simulink model "Simulation_MIMO_MPC_Dreitank_EKF"  (R2022b)
settings: Solver=ode3  StartTime=0.0  StopTime=150  MaxStep=0.01  RelTol=1e-3  EnableMultiTasking=on
PreLoadFcn:
  | A = [0 1;-1 -1];
  | B = [0 ; 1];
  | C = [1 0];
  | 
  | 
  | X0 = [0;0];
  | X_dot0 = [0;0];
  | Y0 = [0;];
  | U0 = [0];
  | 
  | X_AP = X0;
  | U_AP = U0;
  | Y_AP = Y0;
  | X_dot_AP = X_dot0;
undefined symbols (not defined in the file): EKF, MPC, N1, N2, Nu, T_MPC
libraries: UtilLib x1
settings Model: SimulationMode=rapid-accelerator  Creator=Matze  LastModifiedBy=vd818225
settings SolverCC: AlgebraicLoopSolver=TrustRegion
settings DataIOCC: SaveFormat=Array  SignalLoggingSaveFormat=ModelDataLogs  SaveOutput=off  SignalLogging=off  DSMLogging=off  SaveTime=off  ReturnWorkspaceOutputs=off
settings OptimizationCC: ExpressionDepthLimit=2147483647  LifeSpan=inf
settings DebuggingCC: UnderspecifiedInitializationDetection=Classic  MergeDetectMultiDrivingBlocksExec=none  SolverPrmCheckMsg=warning  InheritedTsInSrcMsg=none  FcnCallInpInsideContextMsg=warning  UnconnectedInputMsg=warning  UnconnectedOutputMsg=warning  UnconnectedLineMsg=warning  StateNameClashWarn=warning  SFUnexpectedBacktrackingDiag=warning  SFNoUnconditionalDefaultTransitionDiag=warning  SFExecutionAtInitializationDiag=none  SFMachineParentedDataDiag=warning  ArithmeticOperatorsInVariantConditions=warning
settings HardwareCC: ProdBitPerPointer=32  ProdBitPerSizeT=32  ProdBitPerPtrDiffT=32  ProdLargestAtomicFloat=None  ProdIntDivRoundTo=Undefined  ProdEndianess=Unspecified  ProdWordSize=32  ProdHWDeviceType=32-bit Generic
settings ModelReferenceCC: EnableRefExpFcnMdlSchedulingChecks=on  PropagateSignalLabelsOutOfModel=off
settings SFSimCC: SimUseLocalCustomCode=off  SimParseCustomCode=off  CustomCodeUndefinedFunction=UseInterfaceOnly
settings RTWCC: RTWUseLocalCustomCode=off  DLArmComputeVersion=19.05
settings CodeAppCC: StateflowObjectComments=on
settings GRTTargetCC: TargetLangStandard=C89/C90 (ANSI)  CombineOutputUpdateFcns=off  GRTInterface=on
settings ConfigComp: CovMetricSettings=dw  CovSaveCumulativeToWorkspaceVar=on  CovSaveSingleToWorkspaceVar=on  CovExternalEMLEnable=off

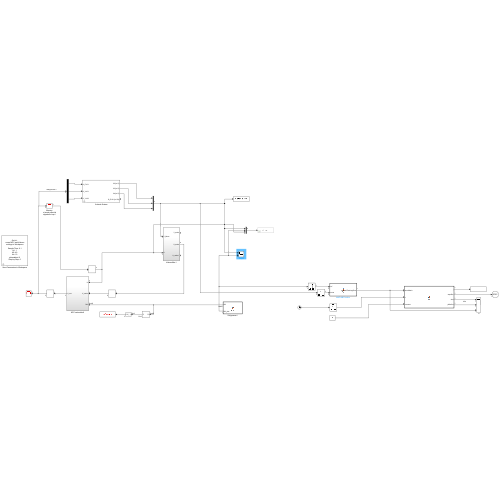
[thumbnail: Simulink's stored preview of the top-level diagram]
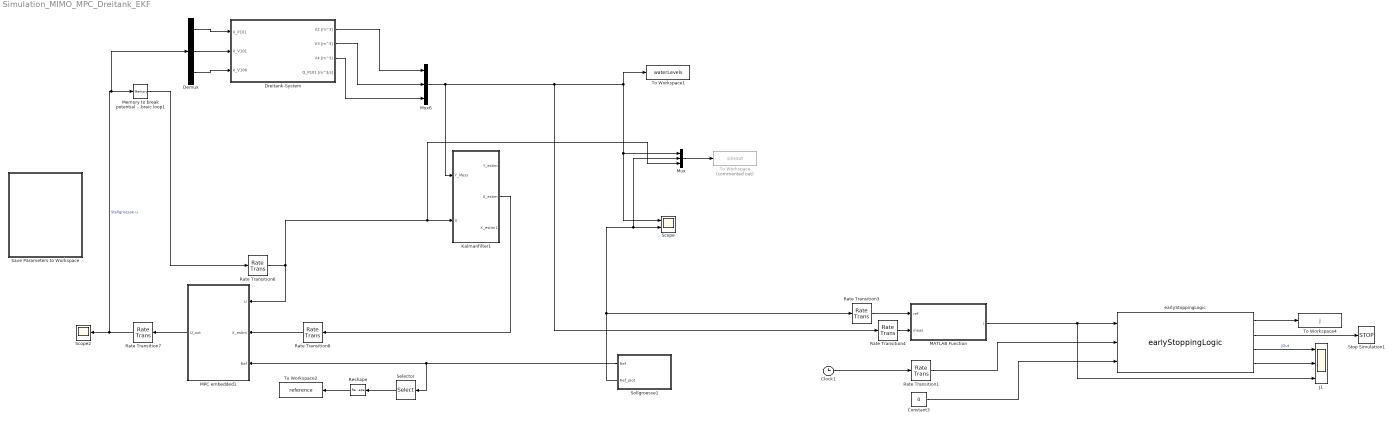
== system Simulation_MIMO_MPC_Dreitank_EKF ==
  Clock1 : Clock
  Constant3 : Constant  Value=0
  Demux : Demux  Outputs=3
  Dreitank-System : Subsystem  mask{B101_Volumen=80*10^-3, B102_Initial_Volumen=8*10^-3, B103_Initial_Volumen=6*10^-3, B104_Initial_Volumen=5*10^-3, Querschnitt_Rohr_B102_B103=600*10^-6, Querschnitt_Rohr_B103_B104=600*10^-6, Flaeche_Behaelter=0.029}
      mask prompts: B101_Volumen "Volumen im Behälter B101 in m^3"; B102_Initial_Volumen "Initialvolumen im Behälter B102 in m^3"; B103_Initial_Volumen "Initialvolumen im Behälter B103 in m^3"; B104_Initial_Volumen "Initialvolumen im Behälter B104 in m^3"; Querschnitt_Rohr_B102_B103 "Rohrquerschnitt zwischen Behälter B102 und B103 in m^2"; Querschnitt_Rohr_B103_B104 "Rohrquerschnitt zwischen Behälter B103 und B104 in m^2"; Flaeche_Behaelter "Fläche der Behälter in m^2"
  J1 : Scope  NumInputPorts=3
  Kalmanfilter1 : Subsystem
  MATLAB Function : MATLAB Function  TreatAsAtomicUnit=on
  MPC embedded1 : Subsystem
  Memory to break potential algrebraic loop1 : Memory
  Mux : Mux  Inputs=3
  Mux6 : Mux  Inputs=3
  Rate Transition1 : RateTransition  OutPortSampleTime=ESSettings.t_obj
  Rate Transition3 : RateTransition  OutPortSampleTime=ESSettings.t_obj
  Rate Transition4 : RateTransition  OutPortSampleTime=ESSettings.t_obj
  Rate Transition6 : RateTransition  OutPortSampleTimeOpt=Inherit  OutPortSampleTime=0.1
  Rate Transition7 : RateTransition  OutPortSampleTimeOpt=Inherit  OutPortSampleTime=0.1
  Rate Transition8 : RateTransition  OutPortSampleTimeOpt=Inherit  OutPortSampleTime=0.1
  Reshape : Reshape
  Save Parameters to Workspace : Subsystem  mask(Double-click open){T_MPC=0.1, N1=1, N2=40, Nu=10, PlotEnabled=off, StepByStep=off}
      mask prompts: T_MPC "Sample Time MPC/Kalman"; PlotEnabled "plot enabled"; StepByStep "Step-by-Step"
      mask init:
      | assignin('base','T_MPC',T_MPC);
      | assignin('base','N1',N1);
      | assignin('base','N2',N2);
      | assignin('base','Nu',Nu);
      | assignin('base','PlotEnabled',PlotEnabled);
      | assignin('base','StepByStep',StepByStep);
      mask Display:
      | disp(['On init: \n saves MPC and Kalman\n settings to Workspace\n\n'    ...
      |         'Sample Time: ' num2str(T_MPC) '\n'...
      |         'N1: ' num2str(N1) '\n'...
      |         'N2: ' num2str(N2) '\n'...
      |         'Nu: ' num2str(Nu) '\n'...
      |         'plotenabled: ' num2str(PlotEnabled) '\n'...
      |         'Step-by-Step: ' num2str(StepByStep) '\n'...
      | ]);
  Scope : Scope  NumInputPorts=2
  Scope2 : Scope
  Selector : Selector  NumberOfDimensions=2  InputPortWidth=3  IndexOptions=Index vector (dialog),Index vector (dialog)  Indices=[1:3],1  OutputSizes=1,1
  Sollgroesse1 : MATLAB Function  TreatAsAtomicUnit=on
  Stop Simulation1 : Stop
  To Workspace : ToWorkspace  Commented=on  VariableName=simout  SaveFormat=Timeseries  SampleTime=-1
  To Workspace1 : ToWorkspace  VariableName=waterLevels  SaveFormat=Structure With Time  SampleTime=0.1
  To Workspace2 : ToWorkspace  VariableName=reference  SaveFormat=Structure With Time  SampleTime=0.1
  To Workspace4 : ToWorkspace  VariableName=j  SaveFormat=Structure With Time  SampleTime=-1
  earlyStoppingLogic : UtilLib/earlyStoppingLogic  SystemSampleTime=-1  VariantActivationTime=update diagram  Latency=0  AutoFrameSizeCalculation=off
  wires:
  Sollgroesse1/1(Ref) -> Selector/1, MPC embedded1/3(Ref)
  Memory to break potential algrebraic loop1/1 -> Rate Transition6/1
  MPC embedded1/1(U_out) -> Rate Transition7/1
  Rate Transition6/1 -> MPC embedded1/1(U), Kalmanfilter1/2(U), Mux/3
  Rate Transition8/1 -> MPC embedded1/2(X_estim)
  Rate Transition7/1 -> Demux/1, Memory to break potential algrebraic loop1/1, Scope2/1  "Stellgroesse u"
  Mux/1 -> To Workspace/1
  Kalmanfilter1/2(X_estim) -> Rate Transition8/1
  Demux/1 -> Dreitank-System/1(U_P101)
  Demux/2 -> Dreitank-System/2("U_V101 ")
  Demux/3 -> Dreitank-System/3(U_V106)
  Dreitank-System/1(V2 [m^3]) -> Mux6/1
  Dreitank-System/2(V3 [m^3]) -> Mux6/2
  Dreitank-System/3(V4 [m^3]) -> Mux6/3
  Selector/1 -> Reshape/1
  Reshape/1 -> To Workspace2/1
  earlyStoppingLogic/4 -> J1/2
  earlyStoppingLogic/1 -> To Workspace4/1
  Rate Transition4/1 -> MATLAB Function/2(meas)
  MATLAB Function/1(j) -> J1/3, earlyStoppingLogic/1
  Rate Transition1/1 -> earlyStoppingLogic/2
  Clock1/1 -> Rate Transition1/1
  earlyStoppingLogic/2 -> Stop Simulation1/1
  Constant3/1 -> earlyStoppingLogic/3
  earlyStoppingLogic/3 -> J1/1  "JOut"
  Mux6/1 -> Kalmanfilter1/1(Y_Mess), Rate Transition4/1, Mux/1, Scope/1, To Workspace1/1
  Rate Transition3/1 -> MATLAB Function/1(ref)
  Sollgroesse1/2(Ref_plot) -> Rate Transition3/1, Mux/2, Scope/2

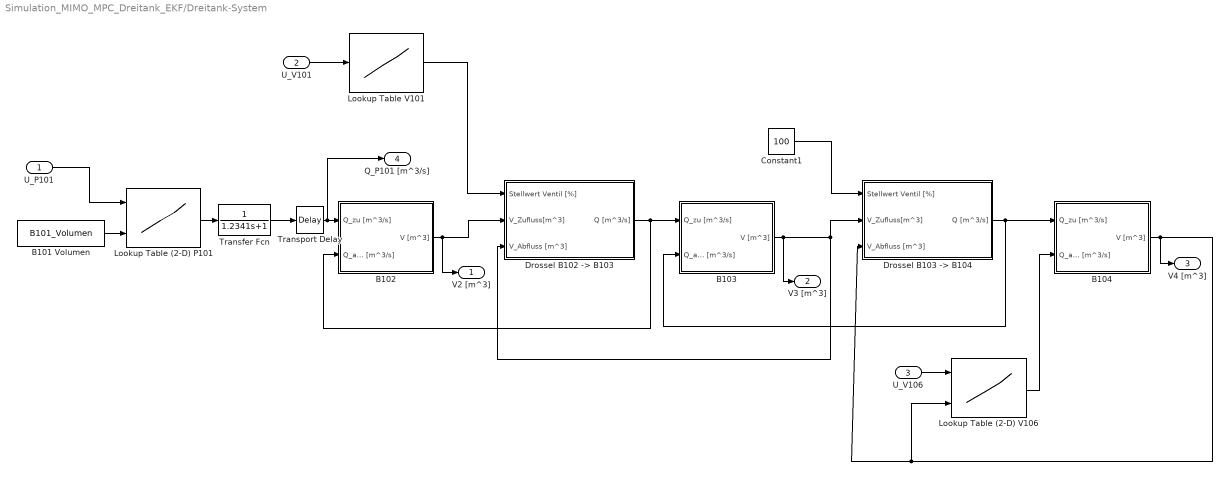
== system Simulation_MIMO_MPC_Dreitank_EKF/Dreitank-System ==
  U_P101 : Inport
  "U_V101 " : Inport  Port=2
  U_V106 : Inport  Port=3
  B101 Volumen : Constant  Value=B101_Volumen  OutDataTypeStr=double
  B102 : Subsystem  mask{Initial_Volumen=B102_Initial_Volumen}
      mask prompts: Initial_Volumen "Initialvolumen"
  B103 : Subsystem  mask{Initial_Volumen=B103_Initial_Volumen}
      mask prompts: Initial_Volumen "Initialvolumen"
  B104 : Subsystem  mask{Initial_Volumen=B104_Initial_Volumen}
      mask prompts: Initial_Volumen "Initialvolumen"
  Constant1 : Constant  Value=100
  "Drossel B102 -> B103" : Subsystem  mask{Querschnitt_Rohr=Querschnitt_Rohr_B102_B103, Flaeche_Behaelter=Flaeche_Behaelter}
      mask prompts: Querschnitt_Rohr "Querschnitt des Rohrs in m^2"; Flaeche_Behaelter "Flaeche_Behaelter in m^2"
  "Drossel B103 -> B104" : Subsystem  mask{Querschnitt_Rohr=Querschnitt_Rohr_B102_B103, Flaeche_Behaelter=Flaeche_Behaelter}
      mask prompts: Querschnitt_Rohr "Querschnitt des Rohrs in m^2"; Flaeche_Behaelter "Flaeche_Behaelter in m^2"
  Lookup Table (2-D) P101 : Lookup2D  RowIndex=[50,55,60,65,70,75,80,85,90,95,100]  ColumnIndex=[40,130]*10^-3  Table=reshape([0,0.0606,0.2450,0.3378,0.4184,0.5002,0.5801,0.6551,0.7138,0.7746,0.8206,0,0.2799,0.3497,0.4278,0.5053,0.5810,0.6481,0.7168,0.7695,0.8350,0.8786]*10^-3,11,2)  LookUpMeth=Interpolation-Use End Values  SaturateOnIntegerOverflow=off  InputSameDT=off
  Lookup Table (2-D) V106 : Lookup2D  RowIndex=[15,20,25,30,35,40,45,50,55,60,65,70,75,80,85]  ColumnIndex=[2,2.8,10]*10^-3  Table=reshape([0,0,0,0,0,0,0,0,0,0,0,0,0,0,0,0,0.032,0.097,0.179,0.262,0.361,0.475,0.604,0.902,1.089,1.318,1.536,1.685,1.853,2.029,0,0.032,0.097,0.179,0.262,0.361,0.475,0.604,0.902,1.089,1.318,1.536,1.685,1.853,2.029]*10^-3,15,3)  LookUpMeth=Interpolation-Use End Values  SaturateOnIntegerOverflow=off  InputSameDT=off
  Lookup Table V101 : Lookup  InputValues=[0,20,25,30,35,40,45,50,55,60,65,70,75,80,85,90,100]  Table=[100,96,90,88,84,76,68,60,49,41,34,27,22,19,16,12,0]  LookUpMeth=Interpolation-Use End Values  SaturateOnIntegerOverflow=off
  Transfer Fcn : TransferFcn  Denominator=[1.2341 1]
  Transport Delay : TransportDelay  DelayTime=1.1
  V2 [m^3] : Outport
  V3 [m^3] : Outport  Port=2
  V4 [m^3] : Outport  Port=3
  Q_P101 [m^3/s] : Outport  Port=4
  wires:
  "Drossel B103 -> B104"/1(Q [m^3/s]) -> B104/1(Q_zu [m^3/s]), B103/2(Q_ab [m^3/s])
  "Drossel B102 -> B103"/1(Q [m^3/s]) -> B102/2(Q_ab [m^3/s]), B103/1(Q_zu [m^3/s])
  B101 Volumen/1 -> Lookup Table (2-D) P101/2
  B103/1(V [m^3]) -> "Drossel B103 -> B104"/2(V_Zufluss[m^3]), "Drossel B102 -> B103"/3(V_Abfluss [m^3]), V3 [m^3]/1
  U_P101/1 -> Lookup Table (2-D) P101/1
  U_V106/1 -> Lookup Table (2-D) V106/1
  Lookup Table V101/1 -> "Drossel B102 -> B103"/1(Stellwert Ventil [%])
  Lookup Table (2-D) V106/1 -> B104/2(Q_ab [m^3/s])
  B102/1(V [m^3]) -> V2 [m^3]/1, "Drossel B102 -> B103"/2(V_Zufluss[m^3])
  "U_V101 "/1 -> Lookup Table V101/1
  B104/1(V [m^3]) -> Lookup Table (2-D) V106/2, "Drossel B103 -> B104"/3(V_Abfluss [m^3]), V4 [m^3]/1
  Constant1/1 -> "Drossel B103 -> B104"/1(Stellwert Ventil [%])
  Transfer Fcn/1 -> Transport Delay/1
  Transport Delay/1 -> Q_P101 [m^3/s]/1, B102/1(Q_zu [m^3/s])
  Lookup Table (2-D) P101/1 -> Transfer Fcn/1

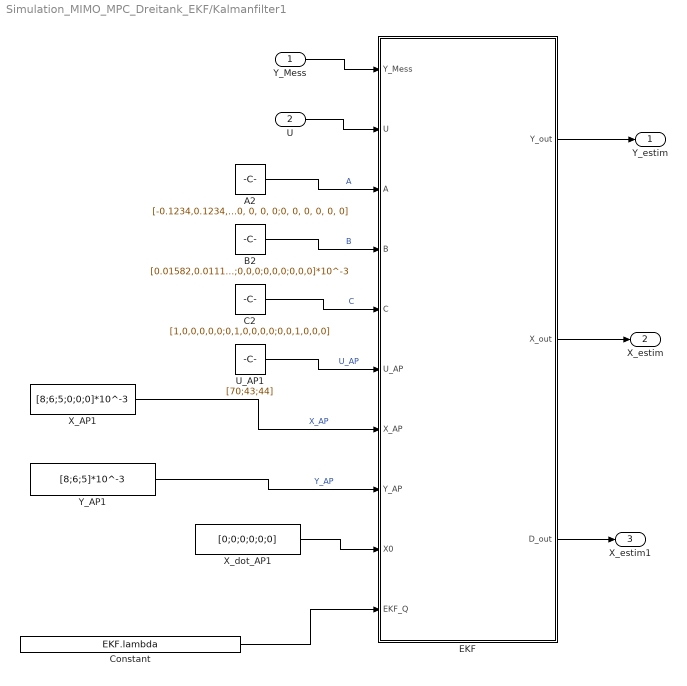
== system Simulation_MIMO_MPC_Dreitank_EKF/Kalmanfilter1 ==
  Y_Mess : Inport
  U : Inport  Port=2
  A2 : Constant  Value=[-0.1234,0.1234,0, 0.025,0,0;0.1234,-0.3702,0.2468, 0,0.025,0 ;0,0.2468,-0.2468, 0,0,0.025; 0, 0, 0, 0, 0, 0;0, 0, 0, 0, 0, 0;0, 0, 0, 0, 0, 0]  VectorParams1D=off
  B2 : Constant  Value=[0.01582,0.01117,0;0,-0.01117,0;0,0,-0.0228;0,0,0;0,0,0;0,0,0]*10^-3  VectorParams1D=off
  C2 : Constant  Value=[1,0,0,0,0,0;0,1,0,0,0,0;0,0,1,0,0,0]  VectorParams1D=off
  Constant : Constant  Value=EKF.lambda
  EKF : MATLAB Function  TreatAsAtomicUnit=on
  U_AP1 : Constant  Value=[70;43;44]  VectorParams1D=off
  X_AP1 : Constant  Value=[8;6;5;0;0;0]*10^-3  VectorParams1D=off
  X_dot_AP1 : Constant  Value=[0;0;0;0;0;0]  VectorParams1D=off
  Y_AP1 : Constant  Value=[8;6;5]*10^-3  VectorParams1D=off
  Y_estim : Outport  VectorParamsAs1DForOutWhenUnconnected=off
  X_estim : Outport  Port=2  VectorParamsAs1DForOutWhenUnconnected=off
  X_estim1 : Outport  Port=3  VectorParamsAs1DForOutWhenUnconnected=off
  wires:
  EKF/1(Y_out) -> Y_estim/1
  U/1 -> EKF/2(U)
  Y_Mess/1 -> EKF/1(Y_Mess)
  EKF/2(X_out) -> X_estim/1
  EKF/3(D_out) -> X_estim1/1
  C2/1 -> EKF/5(C)  "C"
  A2/1 -> EKF/3(A)  "A"
  B2/1 -> EKF/4(B)  "B"
  Y_AP1/1 -> EKF/8(Y_AP)  "Y_AP"
  U_AP1/1 -> EKF/6(U_AP)  "U_AP"
  X_dot_AP1/1 -> EKF/9(X0)
  X_AP1/1 -> EKF/7(X_AP)  "X_AP"
  Constant/1 -> EKF/10(EKF_Q)

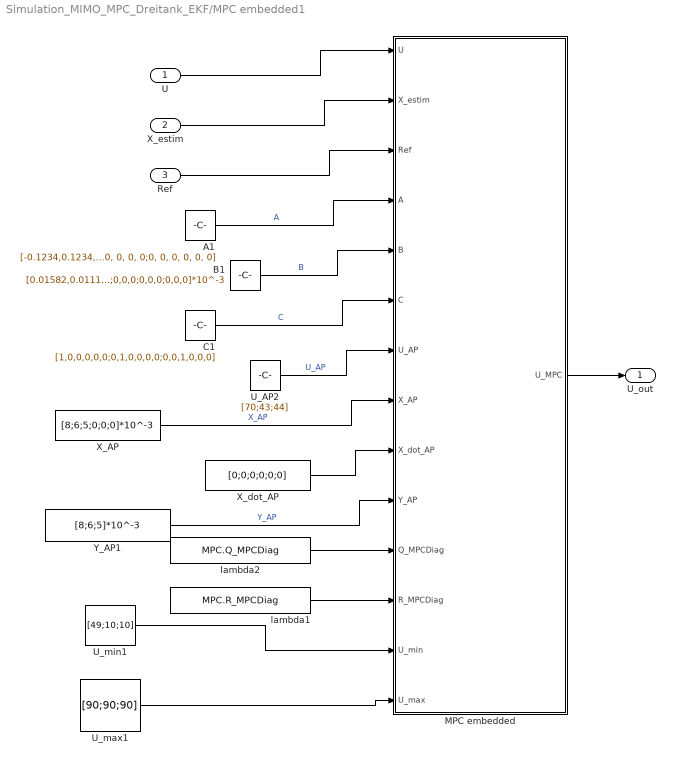
== system Simulation_MIMO_MPC_Dreitank_EKF/MPC embedded1 ==
  U : Inport
  X_estim : Inport  Port=2
  Ref : Inport  Port=3
  A1 : Constant  Value=[-0.1234,0.1234,0, 0.025,0,0;0.1234,-0.3702,0.2468, 0,0.025,0 ;0,0.2468,-0.2468, 0,0,0.025; 0, 0, 0, 0, 0, 0;0, 0, 0, 0, 0, 0;0, 0, 0, 0, 0, 0]  VectorParams1D=off
  B1 : Constant  Value=[0.01582,0.01117,0;0,-0.01117,0;0,0,-0.0228;0,0,0;0,0,0;0,0,0]*10^-3  VectorParams1D=off
  C1 : Constant  Value=[1,0,0,0,0,0;0,1,0,0,0,0;0,0,1,0,0,0]  VectorParams1D=off
  MPC embedded : MATLAB Function  TreatAsAtomicUnit=on
  U_AP2 : Constant  Value=[70;43;44]  VectorParams1D=off
  U_max1 : Constant  Value=[90;90;90]  VectorParams1D=off
  U_min1 : Constant  Value=[49;10;10]  VectorParams1D=off
  X_AP : Constant  Value=[8;6;5;0;0;0]*10^-3  VectorParams1D=off
  X_dot_AP : Constant  Value=[0;0;0;0;0;0]  VectorParams1D=off
  Y_AP1 : Constant  Value=[8;6;5]*10^-3  VectorParams1D=off
  lambda1 : Constant  Value=MPC.R_MPCDiag  VectorParams1D=off
  lambda2 : Constant  Value=MPC.Q_MPCDiag  VectorParams1D=off
  U_out : Outport  VectorParamsAs1DForOutWhenUnconnected=off
  wires:
  B1/1 -> MPC embedded/5(B)  "B"
  C1/1 -> MPC embedded/6(C)  "C"
  lambda2/1 -> MPC embedded/11(Q_MPCDiag)
  Y_AP1/1 -> MPC embedded/10(Y_AP)  "Y_AP"
  U_max1/1 -> MPC embedded/14(U_max)
  A1/1 -> MPC embedded/4(A)  "A"
  X_dot_AP/1 -> MPC embedded/9(X_dot_AP)
  MPC embedded/1(U_MPC) -> U_out/1
  X_AP/1 -> MPC embedded/8(X_AP)  "X_AP"
  U_AP2/1 -> MPC embedded/7(U_AP)  "U_AP"
  X_estim/1 -> MPC embedded/2(X_estim)
  U/1 -> MPC embedded/1(U)
  Ref/1 -> MPC embedded/3(Ref)
  U_min1/1 -> MPC embedded/13(U_min)
  lambda1/1 -> MPC embedded/12(R_MPCDiag)

== system Simulation_MIMO_MPC_Dreitank_EKF/Save Parameters to Workspace ==

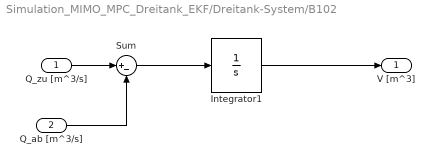
== system Simulation_MIMO_MPC_Dreitank_EKF/Dreitank-System/B102 ==
  Q_zu [m^3/s] : Inport
  Q_ab [m^3/s] : Inport  Port=2
  Integrator1 : Integrator  InitialCondition=Initial_Volumen  LimitOutput=on  UpperSaturationLimit=10*10^-3  LowerSaturationLimit=0  ContinuousStateAttributes='Volumen_B102'
  Sum : Sum  Inputs=|+-
  V [m^3] : Outport
  wires:
  Q_ab [m^3/s]/1 -> Sum/2
  Q_zu [m^3/s]/1 -> Sum/1
  Integrator1/1 -> V [m^3]/1
  Sum/1 -> Integrator1/1

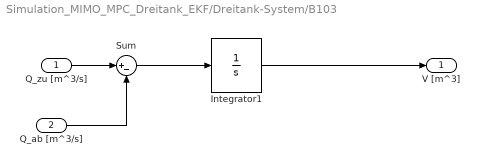
== system Simulation_MIMO_MPC_Dreitank_EKF/Dreitank-System/B103 ==
  Q_zu [m^3/s] : Inport
  Q_ab [m^3/s] : Inport  Port=2
  Integrator1 : Integrator  InitialCondition=Initial_Volumen  LimitOutput=on  UpperSaturationLimit=10*10^-3  LowerSaturationLimit=0  ContinuousStateAttributes='Volumen_B102'
  Sum : Sum  Inputs=|+-
  V [m^3] : Outport
  wires:
  Q_ab [m^3/s]/1 -> Sum/2
  Q_zu [m^3/s]/1 -> Sum/1
  Integrator1/1 -> V [m^3]/1
  Sum/1 -> Integrator1/1

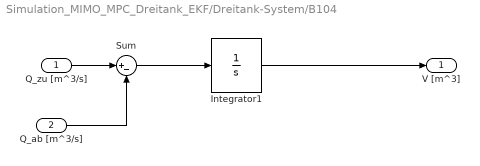
== system Simulation_MIMO_MPC_Dreitank_EKF/Dreitank-System/B104 ==
  Q_zu [m^3/s] : Inport
  Q_ab [m^3/s] : Inport  Port=2
  Integrator1 : Integrator  InitialCondition=Initial_Volumen  LimitOutput=on  UpperSaturationLimit=10*10^-3  LowerSaturationLimit=0  ContinuousStateAttributes='Volumen_B102'
  Sum : Sum  Inputs=|+-
  V [m^3] : Outport
  wires:
  Sum/1 -> Integrator1/1
  Integrator1/1 -> V [m^3]/1
  Q_zu [m^3/s]/1 -> Sum/1
  Q_ab [m^3/s]/1 -> Sum/2

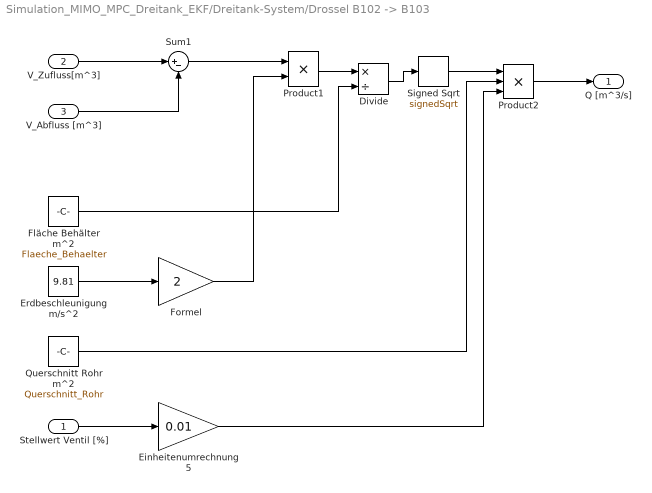
== system Simulation_MIMO_MPC_Dreitank_EKF/Dreitank-System/Drossel B102 -> B103 ==
  Stellwert Ventil [%] : Inport
  V_Zufluss[m^3] : Inport  Port=2
  V_Abfluss [m^3] : Inport  Port=3
  Divide : Product  Inputs=*/
  Einheitenumrechnung 5 : Gain  Gain=0.01
  Erdbeschleunigung m/s^2 : Constant  Value=9.81  OutDataTypeStr=double
  Fläche Behälter m^2 : Constant  Value=Flaeche_Behaelter  OutDataTypeStr=double
  Formel : Gain  Gain=2
  Product1 : Product  RndMeth=Zero
  Product2 : Product  Inputs=3  RndMeth=Zero
  Querschnitt Rohr m^2 : Constant  Value=Querschnitt_Rohr  OutDataTypeStr=double
  Signed Sqrt : Sqrt  Operator=signedSqrt
  Sum1 : Sum  Inputs=|+-
  Q [m^3/s] : Outport
  wires:
  Fläche Behälter m^2/1 -> Divide/2
  Divide/1 -> Signed Sqrt/1
  Product1/1 -> Divide/1
  Formel/1 -> Product1/2
  Sum1/1 -> Product1/1
  V_Abfluss [m^3]/1 -> Sum1/2
  V_Zufluss[m^3]/1 -> Sum1/1
  Product2/1 -> Q [m^3/s]/1
  Einheitenumrechnung 5/1 -> Product2/3
  Stellwert Ventil [%]/1 -> Einheitenumrechnung 5/1
  Querschnitt Rohr m^2/1 -> Product2/2
  Signed Sqrt/1 -> Product2/1
  Erdbeschleunigung m/s^2/1 -> Formel/1

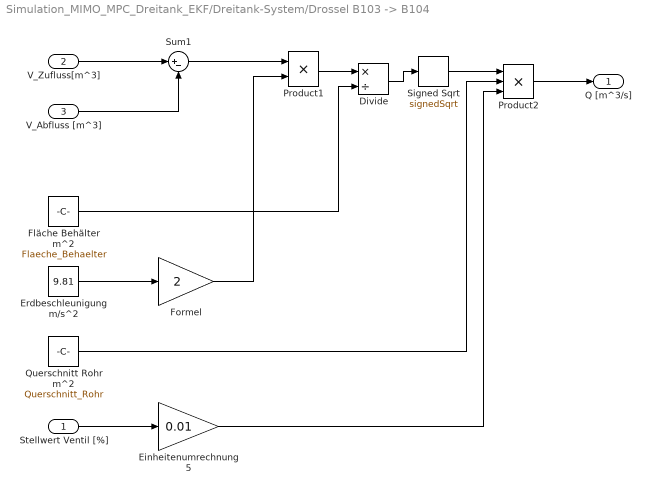
== system Simulation_MIMO_MPC_Dreitank_EKF/Dreitank-System/Drossel B103 -> B104 ==
  Stellwert Ventil [%] : Inport
  V_Zufluss[m^3] : Inport  Port=2
  V_Abfluss [m^3] : Inport  Port=3
  Divide : Product  Inputs=*/
  Einheitenumrechnung 5 : Gain  Gain=0.01
  Erdbeschleunigung m/s^2 : Constant  Value=9.81  OutDataTypeStr=double
  Fläche Behälter m^2 : Constant  Value=Flaeche_Behaelter  OutDataTypeStr=double
  Formel : Gain  Gain=2
  Product1 : Product  RndMeth=Zero
  Product2 : Product  Inputs=3  RndMeth=Zero
  Querschnitt Rohr m^2 : Constant  Value=Querschnitt_Rohr  OutDataTypeStr=double
  Signed Sqrt : Sqrt  Operator=signedSqrt
  Sum1 : Sum  Inputs=|+-
  Q [m^3/s] : Outport
  wires:
  Erdbeschleunigung m/s^2/1 -> Formel/1
  Signed Sqrt/1 -> Product2/1
  Querschnitt Rohr m^2/1 -> Product2/2
  Stellwert Ventil [%]/1 -> Einheitenumrechnung 5/1
  Einheitenumrechnung 5/1 -> Product2/3
  Product2/1 -> Q [m^3/s]/1
  V_Zufluss[m^3]/1 -> Sum1/1
  V_Abfluss [m^3]/1 -> Sum1/2
  Sum1/1 -> Product1/1
  Formel/1 -> Product1/2
  Product1/1 -> Divide/1
  Divide/1 -> Signed Sqrt/1
  Fläche Behälter m^2/1 -> Divide/2

== matlab function Simulation_MIMO_MPC_Dreitank_EKF/MATLAB Function ==
  data: ref input; j output; meas input
function j  = fcn(ref, meas)
j = sum(abs(ref-meas));
end

== matlab function Simulation_MIMO_MPC_Dreitank_EKF/Kalmanfilter1/EKF ==
  settings: updateMethod=DISCRETE  sampleTime=T_MPC
  data: Y_out output; Y_Mess input; U input; A input; B input; C input; U_AP input; X_AP input; Y_AP input; X0 input; EKF_Q input; T_MPC parameter; X_out output; D_out output
function [Y_out, X_out, D_out]  = EKF(Y_Mess,U, A,B,C,U_AP,X_AP, Y_AP, X0,EKF_Q, T_MPC) %#codegen
%%%%%%%%%%%%%%%%%%%%%%%%%%%%%%%%%%%%%%%%%%%%%%%%%%%%%%%%%%%%%%%%%%%%%%%%%%%%%%
% Einfaches Extended Kalmanfilter zur Bestimmung der Zustände am Ende des aktuellen
% Zeitschrittes.
%
% A,B,C: Linearisierte Systemdarstellung
% U_AP, X_AP, Y_AP: Absolutgrößen am Arbeitspunkt (Linearisierung)
% X_dot_AP:         Ableitung des Zustandes am Arbeitspunkt (= 0 für
%                   stationären Arbeitspunkt
% T_MPC:            Abtastrate
%
% Y_Mess: Messgrößenvektor
% X0    : Initialisierungszustand
%
% X_out: Prädierter Zustand am Ende des aktuellen Zeitschrittes
% Y_out: Prädizierte Ausgangsgröße am Ende des aktuellen Zeitschrittes
%
%%%%%%%%%%%%%%%%%%%%%%%%%%%%%%%%%%%%%%%%%%%%%%%%%%%%%%%%%%%%%%%%%%%%%%%%%%%%%%
% Empfohlener Artikel für erste Kalman-Kontakte:
% C. Baumann, "Das Kalman Filter wird 50"
% http://www.convict.lu/htm/rob/Das%20Kalman%20Filter%20wird%2050_v_1.4.pdf
%%%%%%%%%%%%%%%%%%%%%%%%%%%%%%%%%%%%%%%%%%%%%%%%%%%%%%%%%%%%%%%%%%%%%%%%%%%%%%

%%%%%%%%%%%%%%%%%%%%%%%%%%%%%%%%%%%%%%%%%%%%%%%%%%%%%%%%%%%%%%%%%%%%%%%%%%%%%%
%% Zeitkontiunierlich->Zeitdiskret
%%%%%%%%%%%%%%%%%%%%%%%%%%%%%%%%%%%%%%%%%%%%%%%%%%%%%%%%%%%%%%%%%%%%%%%%%%%%%%
[AD, BD, CD]            = Continuous2Discrete(A,B,C,T_MPC);

%%%%%%%%%%%%%%%%%%%%%%%%%%%%%%%%%%%%%%%%%%%%%%%%%%%%%%%%%%%%%%%%%%%%%%%%%%%%%%
%% Initialisierung Zustände im Filter
%%%%%%%%%%%%%%%%%%%%%%%%%%%%%%%%%%%%%%%%%%%%%%%%%%%%%%%%%%%%%%%%%%%%%%%%%%%%%%
persistent X P
if isempty(X)
    X = X0;
    P =  diag(ones(1,size(AD,1)),0 );
end

%%%%%%%%%%%%%%%%%%%%%%%%%%%%%%%%%%%%%%%%%%%%%%%%%%%%%%%%%%%%%%%%%%%%%%%%%%%%%%
%% Umwandlung in Relativgroessen:
%%%%%%%%%%%%%%%%%%%%%%%%%%%%%%%%%%%%%%%%%%%%%%%%%%%%%%%%%%%%%%%%%%%%%%%%%%%%%%
x = X-X_AP;
u = U-U_AP;

%%%%%%%%%%%%%%%%%%%%%%%%%%%%%%%%%%%%%%%%%%%%%%%%%%%%%%%%%%%%%%%%%%%%%%%%%%%%%%
%% Kovarianzmatritzen:
%%%%%%%%%%%%%%%%%%%%%%%%%%%%%%%%%%%%%%%%%%%%%%%%%%%%%%%%%%%%%%%%%%%%%%%%%%%%%%
% Prozessrauschen:
Q = diag(EKF_Q);%diag([1 1 1 10^2 5^2 5^2]);
% Messrauschen:
R = diag(ones(1,size(CD,1)))*10^-2;
%%%%%%%%%%%%%%%%%%%%%%%%%%%%%%%%%%%%%%%%%%%%%%%%%%%%%%%%%%%%%%%%%%%%%%%%%%%%%%%
%% Korrekturschritt
%%%%%%%%%%%%%%%%%%%%%%%%%%%%%%%%%%%%%%%%%%%%%%%%%%%%%%%%%%%%%%%%%%%%%%%%%%%%%%%
MI = CD*P*CD' + R;
K = P*CD'/MI;
deltax = K*(Y_Mess - (Y_AP+CD*x));
x = x+deltax;
P = (eye(size(P)) - K*CD)*P;

%%%%%%%%%%%%%%%%%%%%%%%%%%%%%%%%%%%%%%%%%%%%%%%%%%%%%%%%%%%%%%%%%%%%%%%%%%%%%%%
%% Prädiktionsschritt (hier linear mit aktuellem Modell)
%%%%%%%%%%%%%%%%%%%%%%%%%%%%%%%%%%%%%%%%%%%%%%%%%%%%%%%%%%%%%%%%%%%%%%%%%%%%%%%
x = AD*x+BD*u;   
P = AD*P*AD'+Q;

%%%%%%%%%%%%%%%%%%%%%%%%%%%%%%%%%%%%%%%%%%%%%%%%%%%%%%%%%%%%%%%%%%%%%%%%%%%%%%
%% Umwandlung in Absolutgroessen:
%%%%%%%%%%%%%%%%%%%%%%%%%%%%%%%%%%%%%%%%%%%%%%%%%%%%%%%%%%%%%%%%%%%%%%%%%%%%%%
X = X_AP+x;

%%%%%%%%%%%%%%%%%%%%%%%%%%%%%%%%%%%%%%%%%%%%%%%%%%%%%%%%%%%%%%%%%%%%%%%%%%%%%%%
%% Ausgabe Zustand für nächsten Zeitschritt
%%%%%%%%%%%%%%%%%%%%%%%%%%%%%%%%%%%%%%%%%%%%%%%%%%%%%%%%%%%%%%%%%%%%%%%%%%%%%%%
X_out = X;
Y_out = Y_AP+CD*x;
D_out = P;
end

== matlab function Simulation_MIMO_MPC_Dreitank_EKF/MPC embedded1/MPC embedded ==
  settings: updateMethod=DISCRETE  sampleTime=T_MPC
  data: U input; X_estim input; Ref input; A input; B input; C input; U_AP input; X_AP input; X_dot_AP input; Y_AP input; T_MPC parameter; N1 parameter; N2 parameter; Nu parameter; Q_MPCDiag input; R_MPCDiag input; U_min input; U_max input; U_MPC output
function U_MPC   = MPC_embedded(U,X_estim, Ref, A,B,C,U_AP,X_AP, X_dot_AP, Y_AP,T_MPC, N1, N2, Nu,Q_MPCDiag,R_MPCDiag,U_min, U_max) %#codegen
%%%%%%%%%%%%%%%%%%%%%%%%%%%%%%%%%%%%%%%%%%%%%%%%%%%%%%%%%%%%%%%%%%%%%%%%%
% Gedacht als Referenz-/Beispielimplementierung RT-Skript 
% Im Wesentlichen Umsetzung aus RT-Skript.
% Erweiterung:
%   -Beschränkung Absolutwert Eingangsgroessen
%   -Instationäre Arbeitspunkte möglich
% Verbesserungsvorschläge gerne an RE

%%%%%%%%%%%%%%%%%%%%%%%%%%%%%%%%%%%%%%%%%%%%%%%%%%%%%%%%%%%%%%%%%%%%%%%%%
% Eingangsgrößen:
% U          : Aktueller Absolutert der Stellgröße an der Anlage
% X_estim    : Geschätzer Absolutwert des Zustands am Ende des Zeitschrittes
% Ref        : Sollwertvorgabe (absolut), für jede Regelgröße eine Zeile, passend zum
%              gewählten Prädiktionshorizont
%%%%%%%%%%%%%%%%%%%%%%%%%%%%%%%%%%%%%%%%%%%%%%%%%%%%%%%%%%%%%%%%%%%%%%%%%
% Linearisierte Systembeschreibung:
% A          : Systemmatrix linearisiertes System (kontinuierlich)
% B          : Einfangsmatrix linearisiertes System (kontinuierlich)
% C          : Ausgangsmatrix linearisiertes System (kontinuierlich)
% U_AP       : Stellgröße im Arbeitspunkt
% X_AP       : Zustand im Arbeitspunkt
% X_dot_AP   : Ableitung Zustand im Arbeitspunkt (0 für stationäre Arbeitspunkte) 
% Y_AP       : Ausgang im Arbeitspunkt
%%%%%%%%%%%%%%%%%%%%%%%%%%%%%%%%%%%%%%%%%%%%%%%%%%%%%%%%%%%%%%%%%%%%%%%%%
% MPC-Parameter
% T_MPC      : Abtastschritt
% N1         : unterer Prädiktionshorizont
% N2         : oberer Prädiktionshorizont
% Nu         : Stellhorizont
% lambda_MPC : relative Gewichtung Stellgrößenänderung
% U_min      : Minimalwert Stellgröße (Beschränkung)
% U_max      : Maximalwert Stellgröße (Beschränkung)
%%%%%%%%%%%%%%%%%%%%%%%%%%%%%%%%%%%%%%%%%%%%%%%%%%%%%%%%%%%%%%%%%%%%%%%%%
% Dokumentation und Plot:
% PlotEnabled: Darstellung Werte in Plot
% StepByStep : Pause nach Plot
% Y_doku     : Tatsächlicher Wert Ausgangsgröße (zum Vergleich in Plot)
% currentTime: Simulationszeit für Dokumentation
%%%%%%%%%%%%%%%%%%%%%%%%%%%%%%%%%%%%%%%%%%%%%%%%%%%%%%%%%%%%%%%%%%%%%%%%%


%%%%%%%%%%%%%%%%%%%%%%%%%%%%%%%%%%%%%%%%%%%%%%%%%%%%%%%%%%%%%%%%%%%%%%%%%
%% Berechnung diskrete Zustandsraumdarstellung
%%%%%%%%%%%%%%%%%%%%%%%%%%%%%%%%%%%%%%%%%%%%%%%%%%%%%%%%%%%%%%%%%%%%%%%%%
tic
[AD, BD, CD]        = Continuous2Discrete(A,B,C,T_MPC);

%%%%%%%%%%%%%%%%%%%%%%%%%%%%%%%%%%%%%%%%%%%%%%%%%%%%%%%%%%%%%%%%%%%%%%%%%
%% Generierung MPC-Matritzen
%%%%%%%%%%%%%%%%%%%%%%%%%%%%%%%%%%%%%%%%%%%%%%%%%%%%%%%%%%%%%%%%%%%%%%%%%
[MCA, MCAB,MPhi] = GenerateMPCMatrices(AD,BD,CD, N1, N2, Nu);

%%%%%%%%%%%%%%%%%%%%%%%%%%%%%%%%%%%%%%%%%%%%%%%%%%%%%%%%%%%%%%%%%%%%%%%%%
%% Zwischenvariablen als Hilfestellung 
%%%%%%%%%%%%%%%%%%%%%%%%%%%%%%%%%%%%%%%%%%%%%%%%%%%%%%%%%%%%%%%%%%%%%%%%%
AnzahlStellgroessen = size(BD,2);
AnzahlRegelgroessen = size(CD,1);
Horizontlaenge      = N2-N1+1;

%%%%%%%%%%%%%%%%%%%%%%%%%%%%%%%%%%%%%%%%%%%%%%%%%%%%%%%%%%%%%%%%%%%%%%%%%
%% Umsortieren Referenzggröße auf Vektorform:
%%%%%%%%%%%%%%%%%%%%%%%%%%%%%%%%%%%%%%%%%%%%%%%%%%%%%%%%%%%%%%%%%%%%%%%%%
Ref_vec = reshape(Ref, size(Ref,1)*size(Ref,2),1);

%%%%%%%%%%%%%%%%%%%%%%%%%%%%%%%%%%%%%%%%%%%%%%%%%%%%%%%%%%%%%%%%%%%%%%%%%
%% Umrechnung Absolutgrößen in Größen bezogen auf Arbeitspunkt
%%%%%%%%%%%%%%%%%%%%%%%%%%%%%%%%%%%%%%%%%%%%%%%%%%%%%%%%%%%%%%%%%%%%%%%%%
xk      = X_estim-X_AP;                                 %Zustand
u_km1    = U - U_AP;                                    %Stellgröße aktuell
r       = Ref_vec - repmat(Y_AP,Horizontlaenge,1);      %Sollwert
%%%%%%%%%%%%%%%%%%%%%%%%%%%%%%%%%%%%%%%%%%%%%%%%%%%%%%%%%%%%%%%%%%%%%%%%%
%% Freie Regelgröße (Skript Gl. 10.14) mit Erweiterung um instationären Term
%%%%%%%%%%%%%%%%%%%%%%%%%%%%%%%%%%%%%%%%%%%%%%%%%%%%%%%%%%%%%%%%%%%%%%%%%
%f = MCA*xk + X_estim(4)+MCAB*u_km1 ;
f = MCA*xk +MCAB*u_km1 ;


%%%%%%%%%%%%%%%%%%%%%%%%%%%%%%%%%%%%%%%%%%%%%%%%%%%%%%%%%%%%%%%%%%%%%%%%%
%% Freie Regelabweichung:
%%%%%%%%%%%%%%%%%%%%%%%%%%%%%%%%%%%%%%%%%%%%%%%%%%%%%%%%%%%%%%%%%%%%%%%%%
e = f-r ;

%%%%%%%%%%%%%%%%%%%%%%%%%%%%%%%%%%%%%%%%%%%%%%%%%%%%%%%%%%%%%%%%%%%%%%%%%
%% Wichtungsmatritzen
%%%%%%%%%%%%%%%%%%%%%%%%%%%%%%%%%%%%%%%%%%%%%%%%%%%%%%%%%%%%%%%%%%%%%%%%%
%Q_MPC = eye(AnzahlRegelgroessen*Horizontlaenge);  % Für jeden vorhergesagten Wert des Ausgangs und für jeden Zeitschritt
Q_MPC = diag(repmat([Q_MPCDiag],1,Horizontlaenge));  % Für jeden vorhergesagten Wert des Ausgangs und für jeden Zeitschritt
%R_MPC = eye(AnzahlStellgroessen*Nu)*lambda_MPC;   %Für jeden vorhergesagten Wert der Stellgrößenänderung und für jeden Zeitschritt
R_MPC = diag(repmat([R_MPCDiag],1,Nu));
%%%%%%%%%%%%%%%%%%%%%%%%%%%%%%%%%%%%%%%%%%%%%%%%%%%%%%%%%%%%%%%%%%%%%%%%%
%% Aufstellen Optimierungsproblem
%%%%%%%%%%%%%%%%%%%%%%%%%%%%%%%%%%%%%%%%%%%%%%%%%%%%%%%%%%%%%%%%%%%%%%%%%
% Erstelle Problem der Form:
% Minimiere 1/2*x'*H_qp*x + f_qp'*x unter der Bedingung: A_qp*x <=b_qp
%%%%%%%%%%%%%%%%%%%%%%%%%%%%%%%%%%%%%%%%%%%%%%%%%%%%%%%%%%%%%%%%%%%%%%%%%
H_qp = (MPhi'*Q_MPC'*MPhi+R_MPC);
f_qp =  (e'*Q_MPC*MPhi)';
%%%%%%%%%%%%%%%%%%%%%%%%%%%%%%%%%%%%%%%%%%%%%%%%%%%%%%%%%%%%%%%%%%%%%%%%%
%%%%%%%%%%%%%%%%%%%%%%%%%%%%%%%%%%%%%%%%%%%%%%%%%%%%%%%%%%%%%%%%%%%%%%%%%
% Für Begrenzung (Hier Beispiel Absolutwert Stellgroesse)
% Matrix für Berechnung von Uabs
%%%%%%%%%%%%%%%%%%%%%%%%%%%%%%%%%%%%%%%%%%%%%%%%%%%%%%%%%%%%%%%%%%%%%%%%%
MDiag = zeros(AnzahlStellgroessen*Nu);
for Horiz = 1:Nu
    for Stellg = 1:AnzahlStellgroessen
        for iHoriz = 1:Horiz
            MDiag((Horiz-1)*AnzahlStellgroessen+1+(Stellg-1),...
                (Stellg-1) +1+(iHoriz-1)*AnzahlStellgroessen) = 1;
        end
    end
end
%%%%%%%%%%%%%%%%%%%%%%%%%%%%%%%%%%%%%%%%%%%%%%%%%%%%%%%%%%%%%%%%%%%%%%%%%
A_qp = [MDiag; -MDiag];
b_qp = [repmat(U_max-u_km1-U_AP,Nu,1);repmat(-U_min+u_km1+U_AP,Nu,1)];
%%%%%%%%%%%%%%%%%%%%%%%%%%%%%%%%%%%%%%%%%%%%%%%%%%%%%%%%%%%%%%%%%%%%%%%%%


%%%%%%%%%%%%%%%%%%%%%%%%%%%%%%%%%%%%%%%%%%%%%%%%%%%%%%%%%%%%%%%%%%%%%%%%%
%% Lösung QP-Problem
%%%%%%%%%%%%%%%%%%%%%%%%%%%%%%%%%%%%%%%%%%%%%%%%%%%%%%%%%%%%%%%%%%%%%%%%%
% Es gibt viele Möglichkeiten, das QP-Problem zu lösen. Für die endgültige
% Implementierung auf der Hardware die entsprechenden Verdächtigen fragen
% (Al, Ka, La, etc...)
%%%%%%%%%%%%%%%%%%%%%%%%%%%%%%%%%%%%%%%%%%%%%%%%%%%%%%%%%%%%%%%%%%%%%%%%%
du_optimal = zeros(AnzahlStellgroessen*Nu,1);   %Startwert (hier 0)

%%%%%%%%%%%%%%%%%%%%%%%%%%%%%%%%%%%%%%%%%%%%%%%%%%%%%%%%%%%%%%%%%%%%%%%%%
% Lösung unbschränkt (Direkt lösbar):
%%%%%%%%%%%%%%%%%%%%%%%%%%%%%%%%%%%%%%%%%%%%%%%%%%%%%%%%%%%%%%%%%%%%%%%%%
%%%%%%%%%%%%%%%%%%%%%%%%%%%%%%%%%%%%%%%%%%%%%%%%%%%%%%%%%%%%%%%%%%%%%%%%%
% Alternative: Direkt:
% du_optimal = -  (MPhi'*Q*MPhi+R) \(MPhi'*Q'*e);
%%%%%%%%%%%%%%%%%%%%%%%%%%%%%%%%%%%%%%%%%%%%%%%%%%%%%%%%%%%%%%%%%%%%%%%%%
% Alternative: fminsearch:
% fminsearch kann zur Plausibilisierung verwendet werden, leider nicht
% hier in embedded Matlab, da keine function handles unterstützt sind.
% Befehl kann aber in Kommantozeile ausgeführt werden.
% [du_optimal,fval,~,~] = fminsearch(@(x)(e'*Q*e + x'*(MPhi'*Q'*MPhi+R)*x + 2*e'*Q*MPhi*x),du_optimal);
%%%%%%%%%%%%%%%%%%%%%%%%%%%%%%%%%%%%%%%%%%%%%%%%%%%%%%%%%%%%%%%%%%%%%%%%%

%%%%%%%%%%%%%%%%%%%%%%%%%%%%%%%%%%%%%%%%%%%%%%%%%%%%%%%%%%%%%%%%%%%%%%%%%
% Lösung mit Beschränkung:
%%%%%%%%%%%%%%%%%%%%%%%%%%%%%%%%%%%%%%%%%%%%%%%%%%%%%%%%%%%%%%%%%%%%%%%%%
%%%%%%%%%%%%%%%%%%%%%%%%%%%%%%%%%%%%%%%%%%%%%%%%%%%%%%%%%%%%%%%%%%%%%%%%%
% Alternative: fminsearch:
% fmincon kann zur Plausibilisierung verwendet werden, leider nicht
% hier in embedded Matlab, da keine function handles unterstützt sind.
% Befehl kann aber in Kommantozeile ausgeführt werden.
% du_optimal = fmincon(@(x)(e'*Q*e + x'*H_qp*x + 2*f_qp'*x),zeros(Nu*AnzahlStellgroessen,1),A_qp,b_qp,[],[],[],[],[],optimset('Display', 'off', 'Algorithm', 'active-set'));
%%%%%%%%%%%%%%%%%%%%%%%%%%%%%%%%%%%%%%%%%%%%%%%%%%%%%%%%%%%%%%%%%%%%%%%%%
% Alternative: quadprog:
%coder.extrinsic('quadprog','optimset');
%du_optimal= quadprog(H_qp,f_qp,A_qp,b_qp,[],[],[],[],[],optimset('algorithm','interior-point-convex','Display','off'));
%%%%%%%%%%%%%%%%%%%%%%%%%%%%%%%%%%%%%%%%%%%%%%%%%%%%%%%%%%%%%%%%%%%%%%%%%

%%%%%%%%%%%%%%%%%%%%%%%%%%%%%%%%%%%%%%%%%%%%%%%%%%%%%%%%%%%%%%%%%%%%%%%%%
% Alternative: QPKWIK (aus Matlab MPC Toolbox)
du_optimal  = SolveQP_QPKWIK_wrapper(H_qp,f_qp, A_qp, b_qp);
%%%%%%%%%%%%%%%%%%%%%%%%%%%%%%%%%%%%%%%%%%%%%%%%%%%%%%%%%%%%%%%%%%%%%%%%%


%%%%%%%%%%%%%%%%%%%%%%%%%%%%%%%%%%%%%%%%%%%%%%%%%%%%%%%%%%%%%%%%%%%%%%%%%
%% Ausgabe (erster Wert)
%%%%%%%%%%%%%%%%%%%%%%%%%%%%%%%%%%%%%%%%%%%%%%%%%%%%%%%%%%%%%%%%%%%%%%%%%
uout = u_km1;
for is = 1:AnzahlStellgroessen
    uout(is) = uout(is)+ du_optimal(is);
end
U_MPC = uout + U_AP;
toc
%%%%%%%%%%%%%%%%%%%%%%%%%%%%%%%%%%%%%%%%%%%%%%%%%%%%%%%%%%%%%%%%%%%%%%%%%


%%%%%%%%%%%%%%%%%%%%%%%%%%%%%%%%%%%%%%%%%%%%%%%%%%%%%%%%%%%%%%%%%%%%%%%%%

== matlab function Simulation_MIMO_MPC_Dreitank_EKF/Sollgroesse1 ==
  settings: updateMethod=DISCRETE  sampleTime=T_MPC
  data: N1 parameter; Ref output; N2 parameter; Ref_plot output
function [Ref, Ref_plot] = fcn(N1, N2)
%#codegen
 %Zähler initialisieren
persistent i
if isempty(i)
    i = 1;
end 
%%%%%%%%%%%%%%%%%%%%%%%%%%%%%5
% N1: unterer Stellhorizont
% N2: oberer Stellhorizont
% Ref: Ausgabematrix für MPC
% Ref: Ausgabematrix für MPC

%Generierung Sollgröße für MPC
%Sollgröße für erste Regelgrößen
W1 =  ones(1,500)*1*10^-3;
W2 =  ones(1,500)*1*10^-3;
W3 =  ones(1,500)*1*10^-3;

W1_1 =  ones(1,550)*6*10^-3;
W2_1 =  ones(1,550)*5*10^-3;
W3_1 =  ones(1,550)*4.5*10^-3;

W1_2 =  ones(1,15000)*7*10^-3;
W2_2 =  ones(1,15000)*6*10^-3;
W3_2 =  ones(1,15000)*5*10^-3;
%Optional: Sollgröße für zweite... Regelgröße
%W2 =  [(0:0.1:1) (1:-0.1:0) linspace(0,1,5) linspace(0.5,0,25) linspace(0,1,20)  linspace(1,0,20)];

%WGES: Matrix mit Trajektorie für alle Regelgrößen. Jede Regelgröße bekommt eine Zeile:
%        |-------------------------------------------------------------------------------|
%        | Regelgröße1,Zeitpunkt0 |Regelgröße1,Zeitpunkt1 | Regelgröße1,Zeitpunkt2 | ... |
% WGES = |-------------------------------------------------------------------------------|   
%        | Regelgröße2,Zeitpunkt0 |Regelgröße2,Zeitpunkt1 | Regelgröße2,Zeitpunkt2 | ... |
%        |-------------------------------------------------------------------------------|

%WGES = W1
WGES = [W1 W1_1 W1_2;W2 W2_1 W2_2;W3 W3_1 W3_2];
%WGES = [ W1_1 W1_2; W2_1 W2_2; W3_1 W3_2];

%Relevanten Teil für Prädigketionshorizont aussuchen:
Ref         = WGES(:,(N1:N2)+i+1);   % Um eins verschoben, da der Regler zu Beginn des aktuellen nur auf das Ende des nächsten Zeitschritts zielen kann.
%Ausgabe für Scope (nur aktueller Wert) 
Ref_plot    = WGES(:,i);
 
 
%Zähler hochsetzen
  if N2+i < length(WGES)
     i = i+1;
 end
